simulink model "modelo_FK_trial_1_blocos"  (R2013a)
settings: Solver=ode45  StartTime=0.0  StopTime=1000  RelTol=1e-3
libraries: dspmtrx3 x10, aerolibtransform2 x3, aerolibutil x3, vrlib x2, dspinverses x1
settings Model: Creator=Daniel  LastModifiedBy=Administrator

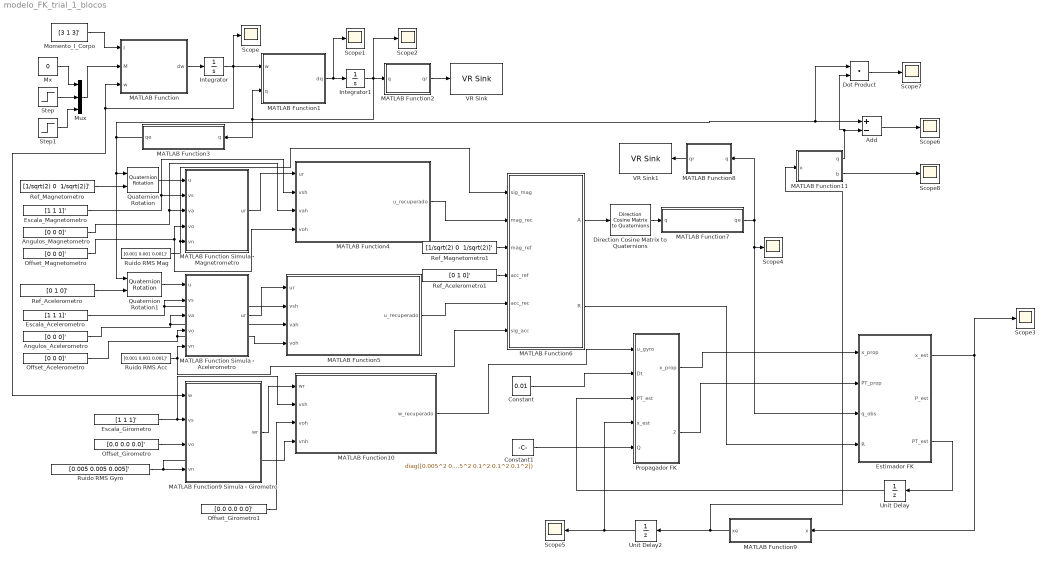
== system modelo_FK_trial_1_blocos ==
  Add : Sum  Inputs=+-
  Angulos_Acelerometro : Constant  Value=[0 0 0]'
  Angulos_Magnetometro : Constant  Value=[0 0 0]'
  Constant : Constant  Value=0.01
  Constant1 : Constant  Value=diag([0.005^2 0.005^2 0.005^2 0.1^2 0.1^2 0.1^2])
  Direction Cosine Matrix to Quaternions : aerolibtransform2/Direction Cosine Matrix  to Quaternions
  Dot Product : DotProduct  InputSameDT=on  OutDataTypeStr=Inherit: Inherit via internal rule
  Escala_Acelerometro : Constant  Value=[1 1 1]'
  Escala_Girometro : Constant  Value=[1 1 1]'
  Escala_Magnetometro : Constant  Value=[1 1 1]'
  Estimador FK : Subsystem  TreatAsAtomicUnit=on  SystemSampleTime=0.01
  Integrator : Integrator  InitialCondition=[0 0 0]
  Integrator1 : Integrator  InitialCondition=[1 0 0 0]
  MATLAB Function : MATLAB Function  TreatAsAtomicUnit=on
  MATLAB Function Simula - Acelerometro : MATLAB Function  TreatAsAtomicUnit=on
  MATLAB Function Simula - Magnetrometro : MATLAB Function  TreatAsAtomicUnit=on
  MATLAB Function1 : MATLAB Function  TreatAsAtomicUnit=on
  MATLAB Function10 : MATLAB Function  TreatAsAtomicUnit=on
  MATLAB Function11 : MATLAB Function  TreatAsAtomicUnit=on
  MATLAB Function2 : MATLAB Function  TreatAsAtomicUnit=on
  MATLAB Function3 : MATLAB Function  TreatAsAtomicUnit=on
  MATLAB Function4 : MATLAB Function  TreatAsAtomicUnit=on
  MATLAB Function5 : MATLAB Function  TreatAsAtomicUnit=on
  MATLAB Function6 : MATLAB Function  TreatAsAtomicUnit=on
  MATLAB Function7 : MATLAB Function  TreatAsAtomicUnit=on
  MATLAB Function8 : MATLAB Function  TreatAsAtomicUnit=on
  MATLAB Function9 : MATLAB Function  TreatAsAtomicUnit=on
  MATLAB Function9 Simula - Girometro : MATLAB Function  TreatAsAtomicUnit=on
  Momento_I_Corpo : Constant  Value=[3 1 3]'
  Mux : Mux  Inputs=3
  Mx : Constant  Value=0
  Offset_Acelerometro : Constant  Value=[0 0 0]'
  Offset_Girometro : Constant  Value=[0.0 0.0 0.0]'
  Offset_Girometro1 : Constant  Value=[0.0 0.0 0.0]'
  Offset_Magnetometro : Constant  Value=[0 0 0]'
  Propagador FK : Subsystem  TreatAsAtomicUnit=on  SystemSampleTime=0.01
  Quaternion Rotation : aerolibutil/Quaternion Rotation
  Quaternion Rotation1 : aerolibutil/Quaternion Rotation
  Ref_Acelerometro : Constant  Value=[0 1 0]'
  Ref_Acelerometro1 : Constant  Value=[0 1 0]'
  Ref_Magnetometro : Constant  Value="[1/sqrt(2) 0  1/sqrt(2)]'"
  Ref_Magnetometro1 : Constant  Value="[1/sqrt(2) 0  1/sqrt(2)]'"
  Ruido RMS Acc : Constant  Value=[0.001 0.001 0.001]'
  Ruido RMS Gyro : Constant  Value=[0.005 0.005 0.005]'
  Ruido RMS Mag : Constant  Value=[0.001 0.001 0.001]'
  Scope{,1..8} (9 alike) : Scope
      Scope2 settings: SaveName=ScopeData2
      Scope3 settings: YMin=-3.25  YMax=1.75  SaveName=ScopeData3  MaxDataPoints=50000
      Scope4 settings: YMin=-1  YMax=1  SaveName=ScopeData4  MaxDataPoints=60000
      Scope5 settings: YMin=-250  YMax=125  SaveName=ScopeData5  MaxDataPoints=50000
      Scope6 settings: YMin=-0.1  YMax=0.11  SaveName=ScopeData6  MaxDataPoints=50000
      Scope7 settings: YMin=-1  YMax=1.75  SaveName=ScopeData7  MaxDataPoints=50000
      Scope8 settings: YMin=-3.25  YMax=1.25  SaveName=ScopeData10  MaxDataPoints=50000
  Step : Step  Time=.1  Before=.2  After=0  SampleTime=0
  Step1 : Step  Time=.1  Before=.02  After=0  SampleTime=0
  Unit Delay : UnitDelay  InitialCondition=diag([100 100 100 100 100 100])  SampleTime=.01
  Unit Delay2 : UnitDelay  InitialCondition=[1 0 0 0 0.1 0.2 0.3]'  SampleTime=.01
  VR Sink : vrlib/VR Sink  InstantiateOnLoad=on  SampleTime=.1  ViewEnable=on  RemoteChange=off  RemoteView=off  FieldsWritten=H.rotation.4.1.1.double  WorldFileName=C:\Users\Administrator\Desktop\Arquivos WRL\cilindro3.wrl  AutoView=off  VideoDimensions=[]  AllowVariableSize=off
  VR Sink1 : vrlib/VR Sink  InstantiateOnLoad=on  SampleTime=.1  ViewEnable=on  RemoteChange=off  RemoteView=off  FieldsWritten=H.rotation.4.1.1.double  WorldFileName=C:\Users\Administrator\Desktop\Arquivos WRL\cilindro4.wrl  AutoView=off  VideoDimensions=[]  AllowVariableSize=off
  wires:
  Momento_I_Corpo/1 -> MATLAB Function/1(I)
  Mux/1 -> MATLAB Function/2(M)
  Mx/1 -> Mux/1
  Step/1 -> Mux/2
  Step1/1 -> Mux/3
  MATLAB Function/1(dw) -> Integrator/1
  Integrator/1 -> MATLAB Function1/1(w), Scope/1, MATLAB Function/3(w), MATLAB Function9 Simula - Girometro/1(w)
  MATLAB Function1/1(dq) -> Integrator1/1, Scope1/1
  Integrator1/1 -> MATLAB Function3/1(q), MATLAB Function1/2(q), Scope2/1, MATLAB Function2/1(q)
  MATLAB Function2/1(qr) -> VR Sink/1
  Quaternion Rotation/1 -> MATLAB Function Simula - Magnetrometro/1(u)
  Quaternion Rotation1/1 -> MATLAB Function Simula - Acelerometro/1(u)
  MATLAB Function3/1(qe) -> Quaternion Rotation/1, Quaternion Rotation1/1, Dot Product/1, Add/1
  Ref_Magnetometro/1 -> Quaternion Rotation/2
  Ref_Acelerometro/1 -> Quaternion Rotation1/2
  Ruido RMS Mag/1 -> MATLAB Function6/1(sig_mag), MATLAB Function Simula - Magnetrometro/5(vn)
  Ruido RMS Acc/1 -> MATLAB Function Simula - Acelerometro/5(vn), MATLAB Function6/6(sig_acc)
  Offset_Magnetometro/1 -> MATLAB Function Simula - Magnetrometro/4(vo), MATLAB Function4/4(voh)
  Escala_Acelerometro/1 -> MATLAB Function Simula - Acelerometro/2(vs), MATLAB Function5/2(vsh)
  Angulos_Acelerometro/1 -> MATLAB Function Simula - Acelerometro/3(va), MATLAB Function5/3(vah)
  Offset_Acelerometro/1 -> MATLAB Function Simula - Acelerometro/4(vo), MATLAB Function5/4(voh)
  MATLAB Function Simula - Magnetrometro/1(ur) -> MATLAB Function4/1(ur)
  MATLAB Function Simula - Acelerometro/1(ur) -> MATLAB Function5/1(ur)
  Escala_Magnetometro/1 -> MATLAB Function Simula - Magnetrometro/2(vs), MATLAB Function4/2(vsh)
  Angulos_Magnetometro/1 -> MATLAB Function Simula - Magnetrometro/3(va), MATLAB Function4/3(vah)
  MATLAB Function5/1(u_recuperado) -> MATLAB Function6/5(acc_rec)
  MATLAB Function4/1(u_recuperado) -> MATLAB Function6/2(mag_rec)
  Ref_Magnetometro1/1 -> MATLAB Function6/3(mag_ref)
  Ref_Acelerometro1/1 -> MATLAB Function6/4(acc_ref)
  MATLAB Function6/1(A) -> Direction Cosine Matrix to Quaternions/1
  MATLAB Function8/1(qr) -> VR Sink1/1
  MATLAB Function9 Simula - Girometro/1(wr) -> MATLAB Function10/1(wr)
  Escala_Girometro/1 -> MATLAB Function10/2(vsh), MATLAB Function9 Simula - Girometro/2(vs)
  Offset_Girometro/1 -> MATLAB Function9 Simula - Girometro/3(vo)
  Direction Cosine Matrix to Quaternions/1 -> MATLAB Function7/1(q)
  Ruido RMS Gyro/1 -> MATLAB Function10/4(vnh), MATLAB Function9 Simula - Girometro/4(vn)
  Propagador FK/2(PT_prop) -> Estimador FK/2(PT_prop)
  MATLAB Function6/2(R) -> Estimador FK/4(R)
  Estimador FK/3(PT_est) -> Unit Delay/1
  Unit Delay/1 -> Propagador FK/3(PT_est)
  MATLAB Function10/1(w_recuperado) -> Propagador FK/1(u_gyro)
  Constant/1 -> Propagador FK/2(Dt)
  Constant1/1 -> Propagador FK/5(Q)
  Unit Delay2/1 -> Scope5/1, Propagador FK/4(x_est)
  MATLAB Function11/1(q) -> Dot Product/2, Add/2
  Add/1 -> Scope6/1
  Dot Product/1 -> Scope7/1
  MATLAB Function11/2(b) -> Scope8/1
  MATLAB Function9/1(xe) -> MATLAB Function11/1(x), Unit Delay2/1
  Estimador FK/1(x_est) -> MATLAB Function9/1(x), Scope3/1
  MATLAB Function7/1(qe) -> MATLAB Function8/1(q), Estimador FK/3(q_obs), Scope4/1
  Offset_Girometro1/1 -> MATLAB Function10/3(voh)
  Propagador FK/1(x_prop) -> Estimador FK/1(x_prop)

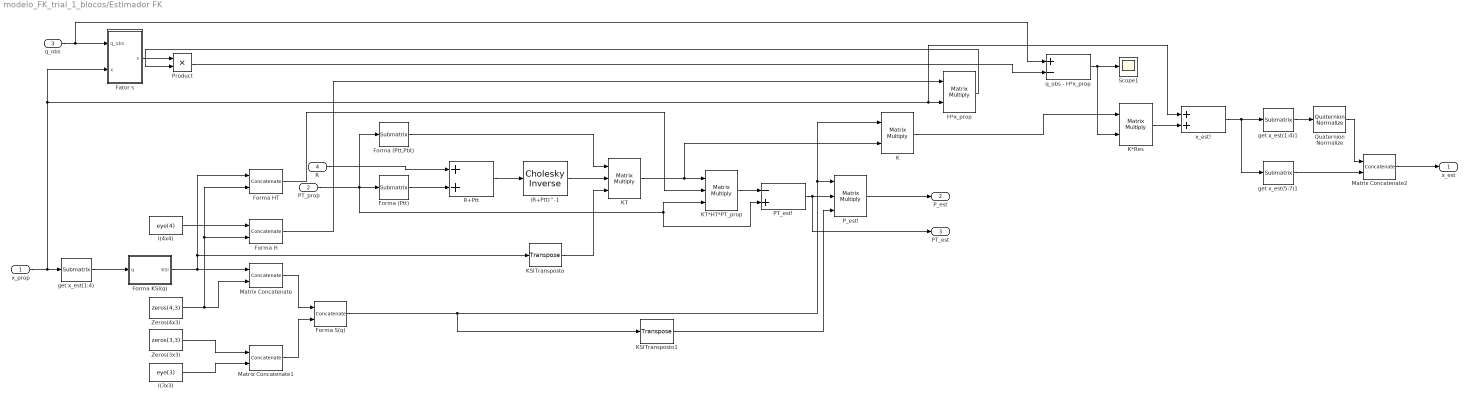
== system modelo_FK_trial_1_blocos/Estimador FK ==
  x_prop : Inport
  PT_prop : Inport  Port=2
  q_obs : Inport  Port=3
  R : Inport  Port=4
  (R+Ptt)^-1 : dspinverses/Cholesky Inverse  errmode=Warning
  Fator s : MATLAB Function  TreatAsAtomicUnit=on
  Forma (Ptt) : dspmtrx3/Submatrix  RowSpan=Range of rows  RowStartMode=First  RowStartIndex=1  RowEndMode=Index  RowEndIndex=3  ColSpan=Range of columns  ColStartMode=First  ColStartIndex=1  ColEndMode=Index  ColEndIndex=3
  Forma (Ptt,Pbt) : dspmtrx3/Submatrix  RowSpan=All rows  RowStartMode=Index  RowStartIndex=4  RowEndMode=Last  RowEndIndex=3  ColSpan=Range of columns  ColStartMode=First  ColStartIndex=1  ColEndMode=Index  ColEndIndex=3
  Forma H : Concatenate  Mode=Multidimensional array  ConcatenateDimension=2
  Forma HT : Concatenate  Mode=Multidimensional array  ConcatenateDimension=2
  Forma KSI(q) : MATLAB Function  TreatAsAtomicUnit=on
  Forma S(q) : Concatenate  Mode=Multidimensional array
  H*x_prop : Product  Multiplication=Matrix(*)
  I(3x3) : Constant  Value=eye(3)
  I(4x4) : Constant  Value=eye(4)
  K : Product  Multiplication=Matrix(*)
  K*Res : Product  Multiplication=Matrix(*)
  KSITransposto : dspmtrx3/Transpose  Hermitian=off  overflowFlag=off
  KSITransposto1 : dspmtrx3/Transpose  Hermitian=off  overflowFlag=off
  KT : Product  Inputs=3  Multiplication=Matrix(*)
  KT*HT*PT_prop : Product  Inputs=3  Multiplication=Matrix(*)
  Matrix Concatenate : Concatenate  Mode=Multidimensional array  ConcatenateDimension=2
  Matrix Concatenate1 : Concatenate  Mode=Multidimensional array  ConcatenateDimension=2
  Matrix Concatenate2 : Concatenate  Mode=Multidimensional array
  PT_est! : Sum  Inputs=-+
  P_est! : Product  Inputs=3  Multiplication=Matrix(*)
  Product : Product
  Quaternion Normalize : aerolibutil/Quaternion Normalize
  R+Ptt : Sum
  Scope1 : Scope
      settings: YMin=-250000  YMax=4e+06  SaveName=ScopeData9  MaxDataPoints=60000
  Zeros(3x3) : Constant  Value=zeros(3,3)
  Zeros(4x3) : Constant  Value=zeros(4,3)
  get x_est(1:4) : dspmtrx3/Submatrix  RowSpan=Range of rows  RowStartMode=Index  RowStartIndex=1  RowEndMode=Index  RowEndIndex=4  ColSpan=All columns  ColStartMode=Index  ColStartIndex=1  ColEndMode=Index  ColEndIndex=1
  get x_est(1:4)1 : dspmtrx3/Submatrix  RowSpan=Range of rows  RowStartMode=Index  RowStartIndex=1  RowEndMode=Index  RowEndIndex=4  ColSpan=All columns  ColStartMode=Index  ColStartIndex=1  ColEndMode=Index  ColEndIndex=1
  get x_est(5:7)1 : dspmtrx3/Submatrix  RowSpan=Range of rows  RowStartMode=Index  RowStartIndex=5  RowEndMode=Index  RowEndIndex=7  ColSpan=All columns  ColStartMode=Index  ColStartIndex=1  ColEndMode=Index  ColEndIndex=1
  q_obs - H*x_prop : Sum  Inputs=+-
  x_est! : Sum
  x_est : Outport
  P_est : Outport  Port=2
  PT_est : Outport  Port=3
  wires:
  q_obs - H*x_prop/1 -> Scope1/1, K*Res/2
  PT_prop/1 -> Forma (Ptt,Pbt)/1, KT*HT*PT_prop/3, PT_est!/2, Forma (Ptt)/1
  Forma KSI(q)/1(KSI) -> Forma HT/1, KSITransposto/1, Matrix Concatenate/1
  Matrix Concatenate1/1 -> Forma S(q)/2
  I(3x3)/1 -> Matrix Concatenate1/2
  Matrix Concatenate2/1 -> x_est/1
  Quaternion Normalize/1 -> Matrix Concatenate2/1
  Forma HT/1 -> KT*HT*PT_prop/2
  KSITransposto1/1 -> P_est!/3
  K/1 -> K*Res/1
  R+Ptt/1 -> (R+Ptt)^-1/1
  Forma (Ptt)/1 -> R+Ptt/2
  x_est!/1 -> get x_est(5:7)1/1, get x_est(1:4)1/1
  get x_est(5:7)1/1 -> Matrix Concatenate2/2
  P_est!/1 -> P_est/1
  R/1 -> R+Ptt/1
  PT_est!/1 -> PT_est/1, P_est!/2
  KT/1 -> K/2, KT*HT*PT_prop/1
  Forma S(q)/1 -> KSITransposto1/1, K/1, P_est!/1
  KT*HT*PT_prop/1 -> PT_est!/1
  get x_est(1:4)/1 -> Forma KSI(q)/1(q)
  Zeros(4x3)/1 -> Forma H/2, Forma HT/2, Matrix Concatenate/2
  Matrix Concatenate/1 -> Forma S(q)/1
  K*Res/1 -> x_est!/2
  (R+Ptt)^-1/1 -> KT/2
  x_prop/1 -> get x_est(1:4)/1, Fator s/2(x), x_est!/1, H*x_prop/2
  get x_est(1:4)1/1 -> Quaternion Normalize/1
  KSITransposto/1 -> KT/3
  Forma (Ptt,Pbt)/1 -> KT/1
  Zeros(3x3)/1 -> Matrix Concatenate1/1
  Forma H/1 -> H*x_prop/1
  q_obs/1 -> q_obs - H*x_prop/1, Fator s/1(q_obs)
  I(4x4)/1 -> Forma H/1
  Fator s/1(s) -> Product/1
  H*x_prop/1 -> Product/2
  Product/1 -> q_obs - H*x_prop/2

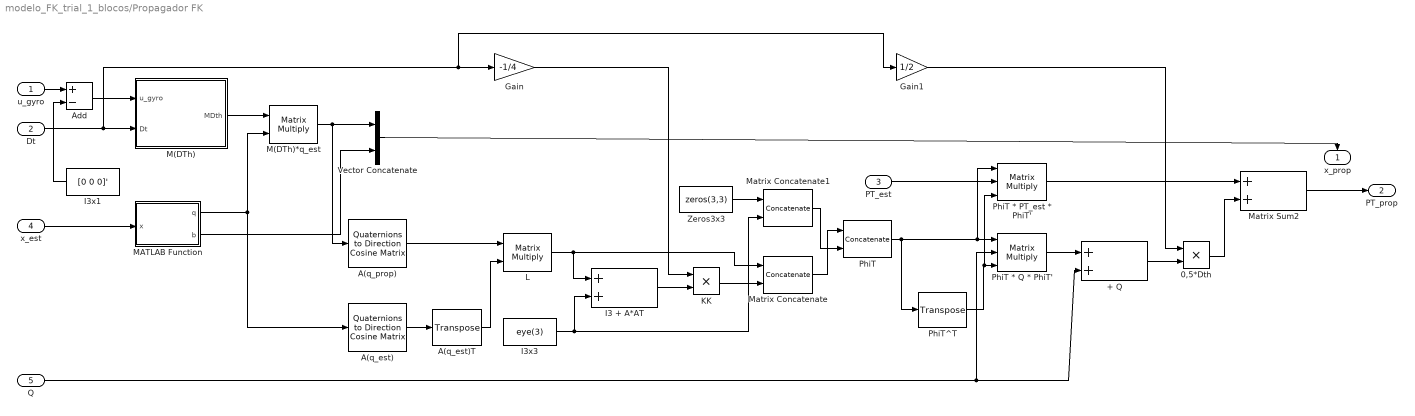
== system modelo_FK_trial_1_blocos/Propagador FK ==
  u_gyro : Inport
  Dt : Inport  Port=2
  PT_est : Inport  Port=3
  x_est : Inport  Port=4
  Q : Inport  Port=5
  + Q : Sum
  0,5*Dth : Product
  A(q_est) : aerolibtransform2/Quaternions to  Direction Cosine Matrix
  A(q_est)T : dspmtrx3/Transpose  Hermitian=off  overflowFlag=off
  A(q_prop) : aerolibtransform2/Quaternions to  Direction Cosine Matrix
  Add : Sum  Inputs=+-
  Gain : Gain  Gain=-1/4
  Gain1 : Gain  Gain=1/2
  I3 + A*AT : Sum
  I3x1 : Constant  Value=[0 0 0]'
  I3x3 : Constant  Value=eye(3)
  KK : Product
  L : Product  Multiplication=Matrix(*)
  M(DTh) : Subsystem
  M(DTh)*q_est : Product  Multiplication=Matrix(*)
  MATLAB Function : MATLAB Function  TreatAsAtomicUnit=on
  Matrix Concatenate : Concatenate  Mode=Multidimensional array  ConcatenateDimension=2
  Matrix Concatenate1 : Concatenate  Mode=Multidimensional array  ConcatenateDimension=2
  Matrix Sum2 : Sum
  PhiT : Concatenate  Mode=Multidimensional array
  "PhiT * PT_est * PhiT' " : Product  Inputs=3  Multiplication=Matrix(*)
  PhiT * Q * PhiT' : Product  Inputs=3  Multiplication=Matrix(*)
  PhiT^T : dspmtrx3/Transpose  Hermitian=off  overflowFlag=off
  Vector Concatenate : Concatenate
  Zeros3x3 : Constant  Value=zeros(3,3)
  x_prop : Outport
  PT_prop : Outport  Port=2
  wires:
  Gain/1 -> KK/1
  MATLAB Function/2(b) -> Vector Concatenate/2
  "PhiT * PT_est * PhiT' "/1 -> Matrix Sum2/1
  L/1 -> Matrix Concatenate/1, I3 + A*AT/1
  x_est/1 -> MATLAB Function/1(x)
  I3 + A*AT/1 -> KK/2
  KK/1 -> Matrix Concatenate/2
  Dt/1 -> Gain/1, Gain1/1, M(DTh)/2(Dt)
  0,5*Dth/1 -> Matrix Sum2/2
  A(q_est)/1 -> A(q_est)T/1
  A(q_prop)/1 -> L/1
  A(q_est)T/1 -> L/2
  Zeros3x3/1 -> Matrix Concatenate1/1
  I3x3/1 -> I3 + A*AT/2, Matrix Concatenate1/2
  M(DTh)/1(MDth) -> M(DTh)*q_est/1
  M(DTh)*q_est/1 -> A(q_prop)/1, Vector Concatenate/1
  PhiT/1 -> PhiT^T/1, "PhiT * PT_est * PhiT' "/1, PhiT * Q * PhiT'/1
  + Q/1 -> 0,5*Dth/2
  Gain1/1 -> 0,5*Dth/1
  PhiT * Q * PhiT'/1 -> + Q/1
  Q/1 -> PhiT * Q * PhiT'/2, + Q/2
  PhiT^T/1 -> "PhiT * PT_est * PhiT' "/3, PhiT * Q * PhiT'/3
  PT_est/1 -> "PhiT * PT_est * PhiT' "/2
  Vector Concatenate/1 -> x_prop/1
  Matrix Sum2/1 -> PT_prop/1
  MATLAB Function/1(q) -> M(DTh)*q_est/2, A(q_est)/1
  Add/1 -> M(DTh)/1(u_gyro)
  u_gyro/1 -> Add/1
  Matrix Concatenate/1 -> PhiT/1
  Matrix Concatenate1/1 -> PhiT/2
  I3x1/1 -> Add/2

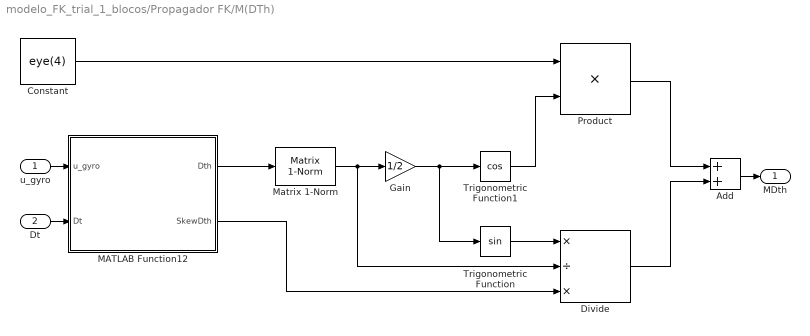
== system modelo_FK_trial_1_blocos/Propagador FK/M(DTh) ==
  u_gyro : Inport
  Dt : Inport  Port=2
  Add : Sum
  Constant : Constant  Value=eye(4)
  Divide : Product  Inputs=*/*
  Gain : Gain  Gain=1/2
  MATLAB Function12 : MATLAB Function  TreatAsAtomicUnit=on
  Matrix 1-Norm : dspmtrx3/Matrix  1-Norm  outputDataTypeStr=Inherit: Same as accumulator  outputLastDataTypeStr=Inherit: Same as accumulator  outputMin=[]  outputMax=[]  roundingMode=Floor  overflowMode=off
  Product : Product
  Trigonometric Function : Trigonometry
  Trigonometric Function1 : Trigonometry  Operator=cos
  MDth : Outport
  wires:
  Product/1 -> Add/1
  MATLAB Function12/2(SkewDth) -> Divide/3
  Gain/1 -> Trigonometric Function/1, Trigonometric Function1/1
  MATLAB Function12/1(Dth) -> Matrix 1-Norm/1
  Matrix 1-Norm/1 -> Divide/2, Gain/1
  Trigonometric Function1/1 -> Product/2
  Trigonometric Function/1 -> Divide/1
  Constant/1 -> Product/1
  Divide/1 -> Add/2
  u_gyro/1 -> MATLAB Function12/1(u_gyro)
  Add/1 -> MDth/1
  Dt/1 -> MATLAB Function12/2(Dt)

== matlab function modelo_FK_trial_1_blocos/MATLAB Function1 ==
  data: w input; dq output; q input
function dq = cinematica(w,q)
%#eml
wx = w(1);
wy = w(2);
wz = w(3);

q = q/norm(q);

qteta = q(1);
qx = q(2);
qy = q(3);
qz = q(4);

W = [0 -wx -wy -wz; wx 0 wz -wy; wy -wz 0 wx; wz wy -wx 0];
%W=[0 wz -wy wx; -wz 0 wx wy; wy -wx 0 wz; -wx -wy -wz 0];
dq=0.5*W*[qteta qx qy qz]';

== matlab function modelo_FK_trial_1_blocos/MATLAB Function ==
  data: I input; dw output; M input; w input
function dw  = Eq_Euler(I,M,w)
%#eml
wx = w(1);
wy = w(2);
wz = w(3);

Ix = I(1);
Iy = I(2);
Iz = I(3);

Mx = M(1);
My = M(2);
Mz = M(3);

dwx = (Mx - wy*wz*(Iz - Iy))/Ix;
dwy = (My - wx*wz*(Ix - Iz))/Iy;
dwz = (Mz - wx*wy*(Iy - Ix))/Iz;

dw=[dwx dwy dwz]';

== matlab function modelo_FK_trial_1_blocos/MATLAB Function2 ==
  data: q input; qr output
function qr = ajusta_q(q)
%#eml

q = q/(norm(q));
v = [q(2) q(3) q(4)] / norm([q(2) q(3) q(4)]);
ang = acos(q(1))*2;

qr = [v ang];

== matlab function modelo_FK_trial_1_blocos/MATLAB Function3 ==
  data: q input; qe output
function qe = tira_redundancia(q)
qe = zeros(4,1);
%#eml

if q(1)<0.0
    qe = -q;
else
    qe = q;
end

== matlab function modelo_FK_trial_1_blocos/MATLAB Function Simula - Magnetrometro ==
  data: u input; ur output; vs input; va input; vo input; vn input
function ur = triad_model(u,vs,va,vo,vn)
%#eml

rho = va(1);
phi = va(2);
lambda = va(3);

S = diag(vs);
T = [1 0 0; sin(rho) cos(rho) 0;...
    sin(phi)*cos(lambda) sin(lambda)*cos(phi) cos(phi)*cos(lambda)];

ur = S*T*u + vo + vn*randn;

== matlab function modelo_FK_trial_1_blocos/MATLAB Function Simula - Acelerometro ==
  data: u input; ur output; vs input; va input; vo input; vn input
function ur = triad_model(u,vs,va,vo,vn)
%#eml

rho = va(1);
phi = va(2);
lambda = va(3);

S = diag(vs);
T = [1 0 0; sin(rho) cos(rho) 0;...
    sin(phi)*cos(lambda) sin(lambda)*cos(phi) cos(phi)*cos(lambda)];

ur = S*T*u + vo + vn*randn;

== matlab function modelo_FK_trial_1_blocos/MATLAB Function4 ==
  data: ur input; u_recuperado output; vsh input; vah input; voh input
function u_recuperado = inv_triad_model(ur,vsh,vah,voh)
%#eml

rho = vah(1);
phi = vah(2);
lambda = vah(3);

T_inv = [1 0 0; -tan(rho) 1/cos(rho) 0;...
    tan(rho)*tan(lambda)-tan(phi) -tan(lambda)/cos(rho) 1/(cos(lambda)*cos(phi))];
S_inv = inv(diag(vsh));

u_recuperado = T_inv*S_inv*(ur - voh);

== matlab function modelo_FK_trial_1_blocos/MATLAB Function5 ==
  data: ur input; u_recuperado output; vsh input; vah input; voh input
function u_recuperado = inv_triad_model(ur,vsh,vah,voh)
%#eml

rho = vah(1);
phi = vah(2);
lambda = vah(3);

T_inv = [1 0 0; -tan(rho) 1/cos(rho) 0;...
    tan(rho)*tan(lambda)-tan(phi) -tan(lambda)/cos(rho) 1/(cos(lambda)*cos(phi))];
S_inv = inv(diag(vsh));

u_recuperado = T_inv*S_inv*(ur - voh);

== matlab function modelo_FK_trial_1_blocos/MATLAB Function6 ==
  data: sig_mag input; A output; mag_rec input; mag_ref input; acc_ref input; acc_rec input; sig_acc input; R output
function [A,R] = TRIAD(sig_mag,mag_rec,mag_ref,acc_ref,acc_rec,sig_acc)

% ========== Função de Determinação de Atitude ===========
% ========== Algoritmo TRIAD ===========
% Os parâmetros de Entrada são:
% V1 : vetor de referência V1
V1 = acc_ref;
% V2 : vetor de referência V2
V2 = mag_ref;
% W1 : vetor de observação W1
W1 = acc_rec;
% W2 : vetor de observação W2
W2 = mag_rec;
% SigTo1 : desvio padrão das observação do Acelerômetro
SigTot1 = sig_mag(1);
% SigTo2 : desvio padrão das observação do Magnetômetro
SigTot2 = sig_acc(1);

% ========================================================
% Os parâmetros de Retorno são:
% A : matriz de atitude
% P : Covariância da atitude
% ========================================================
% --- Obtendo a Tríade de Referência
r1 = V1/norm(V1);
r2 = cross(V1,V2); % função do produto vetorial
r2 = r2 / norm(r2);
r3 = cross(r1,r2);
% --- Montando a Matriz de Referência
Mref = [r1 r2 r3];
% --- Obtendo a tríade de observação
s1 = W1/norm(W1);
s2 = cross(W1,W2);
s2 = s2 / norm(s2);
s3 = cross(s1,s2);
% --- Montando a Matriz de Observação
Mobs = [s1 s2 s3];
% --- Atitude pelo TRIAD
A = Mobs * Mref';
%--------------------------------------------------------------------------
% Obtendo a covariância da atitude (P = P + AP AT)
R = SigTot1^2 * eye(3) + ...
    (1/norm(cross(W1,W2)))^2 * (SigTot1^2* (W1'*W2) * (W1*W2' + W2*W1')...
    + (SigTot2^2 - SigTot1^2)*W1*W1');

%--------------------------------------------------------------------------

== matlab function modelo_FK_trial_1_blocos/MATLAB Function7 ==
  data: q input; qe output
function qe = tira_redundancia(q)
qe = zeros(4,1);
%#eml

if q(1)<0.0
    qe = -q;
else
    qe = q;
end

== matlab function modelo_FK_trial_1_blocos/MATLAB Function8 ==
  data: q input; qr output
function qr = ajusta_q(q)
%#eml

q = q/(norm(q));
v = [q(2) q(3) q(4)] / norm([q(2) q(3) q(4)]);
ang = acos(q(1))*2;

qr = [v ang];

== matlab function modelo_FK_trial_1_blocos/MATLAB Function9 Simula - Girometro ==
  data: w input; wr output; vs input; vo input; vn input
function wr = gyro_model(w,vs,vo,vn)
%#eml

S = diag(vs);

wr = S*w + vo + vn*randn;

== matlab function modelo_FK_trial_1_blocos/MATLAB Function10 ==
  data: wr input; w_recuperado output; vsh input; voh input; vnh input
function w_recuperado = inv_gyro_model(wr,vsh,voh,vnh)
%#eml

S_inv = inv(diag(vsh));

w_recuperado = S_inv*(wr - voh);

== matlab function modelo_FK_trial_1_blocos/MATLAB Function9 ==
  data: x input; xe output
function xe = tira_redundancia(x)
q = x(1:4,1);

if q(1)<0.0
    qe = -q;
else
    qe = q;
end

xe = [qe; x(5:7,1)];

== matlab function modelo_FK_trial_1_blocos/MATLAB Function11 ==
  data: x input; q output; b output
function [q,b] = separa(x)
q = x(1:4,1);
b = x(5:7,1);
end

== matlab function modelo_FK_trial_1_blocos/Propagador FK/M(DTh)/MATLAB Function12 ==
  data: u_gyro input; Dth output; Dt input; SkewDth output
function [Dth,SkewDth] = Delta_Theta(u_gyro,Dt)
Dth = u_gyro * Dt;

dx = Dth(1);
dy = Dth(2);
dz = Dth(3);

SkewDth = [0 -dx -dy -dz;
           dx 0 dz -dy;
           dy -dz 0 dx;
           dz dy -dx 0];
%SkewDth = [0 Dth(3) -Dth(2) Dth(1);
%           -Dth(3) 0 Dth(1) Dth(2);
%           Dth(2) -Dth(1) 0 Dth(3);
%           -Dth(1) -Dth(2) -Dth(3) 0];       
end

== matlab function modelo_FK_trial_1_blocos/Estimador FK/Forma KSI(q) ==
  data: q input; KSI output
function KSI = Forma_KSI(q)
qa = q(1);
qx = q(2);
qy = q(3);
qz = q(4);

KSI = [ qa -qz  qy;
        qz  qa -qx;
       -qy  qx  qa;
       -qx -qy -qz];
end

== matlab function modelo_FK_trial_1_blocos/Propagador FK/MATLAB Function ==
  data: x input; q output; b output
function [q,b] = separa(x)
q = x(1:4,1);
b = x(5:7,1);
end

== matlab function modelo_FK_trial_1_blocos/Estimador FK/Fator s ==
  data: q_obs input; s output; x input
function s = Fator_s(q_obs,x)
q_prop = x(1:4,1);
s = dot(q_obs,q_prop) / norm(dot(q_obs,q_prop));
end
